simulink model "uwb_1"  (R2025a)
settings: Solver=VariableStepAuto  StartTime=0.0  StopTime=5e-08  RelTol=1e-3
undefined symbols (not defined in the file or in its folder): dspblkCoreblockFVToolHelper, gcbh
libraries: commdigbbndpm3 x2, dspfiltersrcs x2, dspsigops x2, simulink_extras x1, dspfdesign x1, simulink x1, commrfcorlib x1
settings Model: Creator=IWMAI  LastModifiedBy=IWMAI

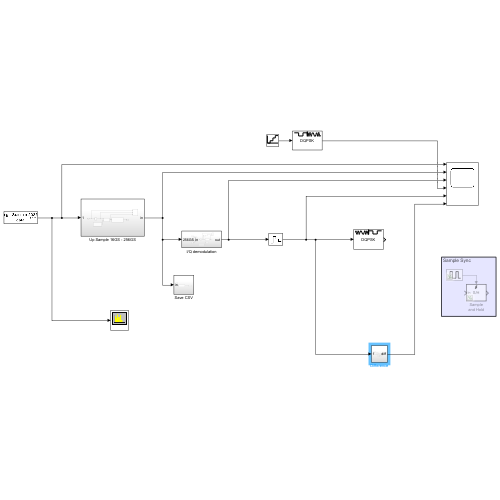
[thumbnail: Simulink's stored preview of the top-level diagram]
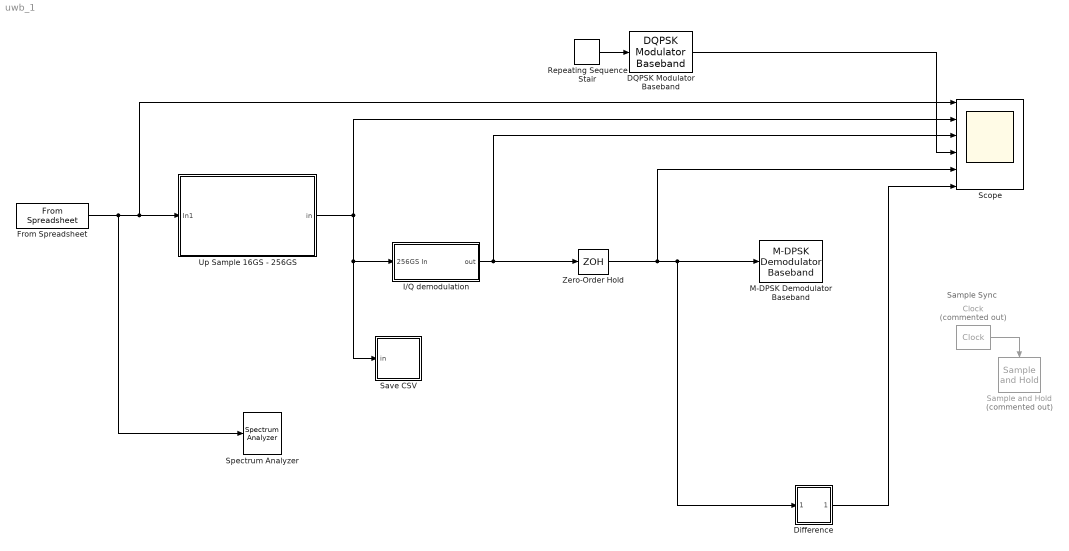
== system uwb_1 ==
  note: Sample Sync
  Clock : simulink_extras/Flip Flops/Clock  Commented=on  period=512.95 / 256e9
  DQPSK Modulator Baseband : commdigbbndpm3/DQPSK Modulator Baseband  InType=Integer  Enc=Gray  Ph=pi/4  outDtype=double
  Difference : Subsystem
  From Spreadsheet : FromSpreadsheet  FileName=C:\Users\IWMAI\University of Toronto\Yu Huang - Summer-2025-sharted\Yongkang\v3_250617\csv\data.csv  SheetName=data  OutDataTypeStr=double  SampleTime=6.25e-11
  I/Q demodulation : Subsystem
  M-DPSK Demodulator Baseband : commdigbbndpm3/M-DPSK Demodulator Baseband  M=4  OutType=Integer  Dec=Gray  Ph=pi/8  outDtype1=Inherit via internal rule  outDtype2=Inherit via internal rule
  Repeating Sequence Stair : simulink/Sources/Repeating Sequence Stair  OutValues=[0 1 2 3].'  tsamp=512.95 / 256e9  OutMin=[]  OutMax=[]  OutDataTypeStr=double  OutputDataTypeScalingMode=double  OutDataType=fixdt(0,8)  ConRadixGroup=Best Precision: Vector-wise  OutScaling=2^-12
  Sample and Hold : dspsigops/Sample and Hold  Commented=on  trig=Rising edge  initCond=0  latchinput=off
  Save CSV : Subsystem
  Scope : Scope  NumInputPorts=6
      settings: ActiveDisplayYMinimum=-0.1766463393208148  ActiveDisplayYMaximum=0.16150855826432609
  Spectrum Analyzer : SpectrumAnalyzer  WindowPosition=[624.000000,326.000000,800.000000,500.000000,]  ScopeFrameLocation=window  WindowInvariantSamplesPerUpdate=on  YLimits=[-72.7658 4.4718]
      settings: OpenAtSimulationStart=off
  Up Sample 16GS - 256GS : Subsystem
  Zero-Order Hold : ZeroOrderHold  SampleTime=512.95 / 256e9
  wires:
  From Spreadsheet/1 -> Spectrum Analyzer/1, Up Sample 16GS - 256GS/1(In1), Scope/1
  Up Sample 16GS - 256GS/1(in) -> Save CSV/1(in), I/Q demodulation/1(256GS In), Scope/2
  I/Q demodulation/1(out) -> Zero-Order Hold/1, Scope/3
  Zero-Order Hold/1 -> Scope/5, Difference/1(In1), M-DPSK Demodulator Baseband/1
  Clock/1 -> Sample and Hold/Trigger
  Repeating Sequence Stair/1 -> DQPSK Modulator Baseband/1
  DQPSK Modulator Baseband/1 -> Scope/4
  Difference/1(diff) -> Scope/6

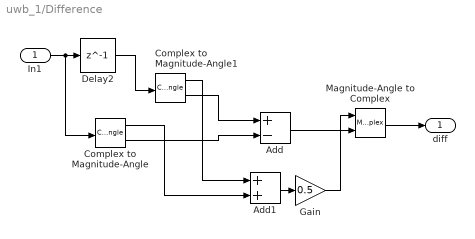
== system uwb_1/Difference ==
  In1 : Inport
  Add : Sum  Inputs=+-
  Add1 : Sum
  Complex to Magnitude-Angle : ComplexToMagnitudeAngle
  Complex to Magnitude-Angle1 : ComplexToMagnitudeAngle
  Delay2 : Delay  DelayLength=1
  Gain : Gain  Gain=0.5
  Magnitude-Angle to Complex : MagnitudeAngleToComplex
  diff : Outport
  wires:
  Gain/1 -> Magnitude-Angle to Complex/1
  Complex to Magnitude-Angle1/2 -> Add/1
  Add1/1 -> Gain/1
  Add/1 -> Magnitude-Angle to Complex/2
  Complex to Magnitude-Angle/2 -> Add/2
  Magnitude-Angle to Complex/1 -> diff/1
  Complex to Magnitude-Angle/1 -> Add1/2
  Complex to Magnitude-Angle1/1 -> Add1/1
  Delay2/1 -> Complex to Magnitude-Angle1/1
  In1/1 -> Delay2/1, Complex to Magnitude-Angle/1

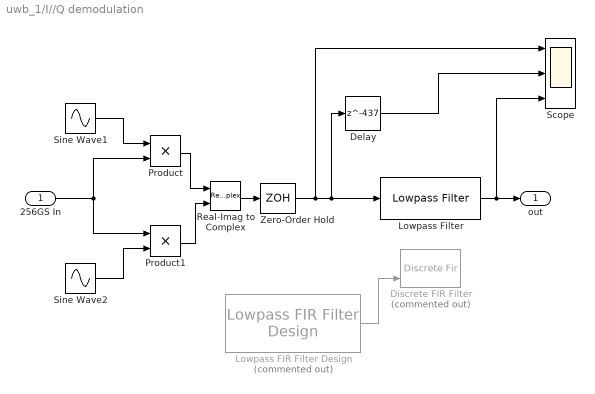
== system uwb_1/I//Q demodulation ==
  256GS In : Inport
  Delay : Delay  DelayLength=437
  Discrete FIR Filter : DiscreteFir  Commented=on  LoadFcn=dspblkCoreblockFVToolHelper(gcbh,'load');  CoefSource=Input port
      settings: CopyFcn=dspblkCoreblockFVToolHelper(gcbh,'copy');  DeleteFcn=dspblkCoreblockFVToolHelper(gcbh,'close');  ModelCloseFcn=dspblkCoreblockFVToolHelper(gcbh,'close');  PreSaveFcn=dspblkCoreblockFVToolHelper(gcbh,'presave');  PostSaveFcn=dspblkCoreblockFVToolHelper(gcbh,'postsave');  CloseFcn=dspblkCoreblockFVToolHelper(gcbh,'close');  InputPortMap=u0,u1
  Lowpass FIR Filter Design : dspfiltersrcs/Lowpass FIR Filter Design  Commented=on  SmoothParameters=off  SmoothingFactor=0.6  FilterOrderPort=off  FilterOrder=100  MaxOrder=100  CutoffFrequencyPort=off  CutoffFrequency=1/256e9  Window=Hann  SidelobeAttenuationPort=off  SidelobeAttenuation=60  KaiserWindowParameterPort=off  KaiserWindowParameter=.5  OutputDataType=double  SampleTime=1/256e9  SimulateUsing=Interpreted execution
      settings: LibrarySourceBlock=dspfdesign/Lowpass FIR Filter Design
  Lowpass Filter : dspfdesign/Lowpass Filter  FilterType=FIR  DesignForMinimumOrder=on  FilterOrder=50  PassbandFrequency=1/128  StopbandFrequency=1/64  PassbandRipple=0.1  StopbandAttenuation=80  SampleRateMode=Use normalized frequency (0 to 1)  SampleRate=44100  SimulateUsing=Interpreted execution  roundingMode=Floor  coeffsDataTypeStr=fixdt(1,16)
  Product : Product
  Product1 : Product
  Real-Imag to Complex : RealImagToComplex
  Scope : Scope  NumInputPorts=3
      settings: ActiveDisplayYMinimum=-6.0977483388597946  ActiveDisplayYMaximum=7.578935112423169  DataLoggingVariableName=ScopeData2
  Sine Wave1 : Sin  Frequency=2 * pi * 3.75e9  Phase=pi/2  SampleTime=0
  Sine Wave2 : Sin  Frequency=2 * pi * 3.75e9  SampleTime=0
  Zero-Order Hold : ZeroOrderHold  SampleTime=1/256e9
  out : Outport
  wires:
  256GS In/1 -> Product/2, Product1/1
  Sine Wave2/1 -> Product1/2
  Sine Wave1/1 -> Product/1
  Product/1 -> Real-Imag to Complex/1
  Product1/1 -> Real-Imag to Complex/2
  Lowpass FIR Filter Design/1 -> Discrete FIR Filter/2
  Lowpass Filter/1 -> Scope/3, out/1
  Real-Imag to Complex/1 -> Zero-Order Hold/1
  Zero-Order Hold/1 -> Scope/1, Delay/1, Lowpass Filter/1
  Delay/1 -> Scope/2

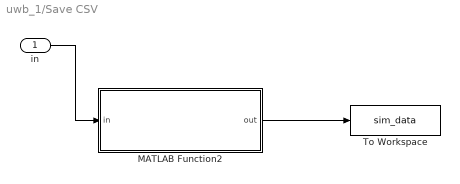
== system uwb_1/Save CSV ==
  in : Inport
  MATLAB Function2 : MATLAB Function  TreatAsAtomicUnit=on
  To Workspace : ToWorkspace  VariableName=sim_data  SaveFormat=Timeseries  SampleTime=-1
  wires:
  MATLAB Function2/1(out) -> To Workspace/1
  in/1 -> MATLAB Function2/1(in)

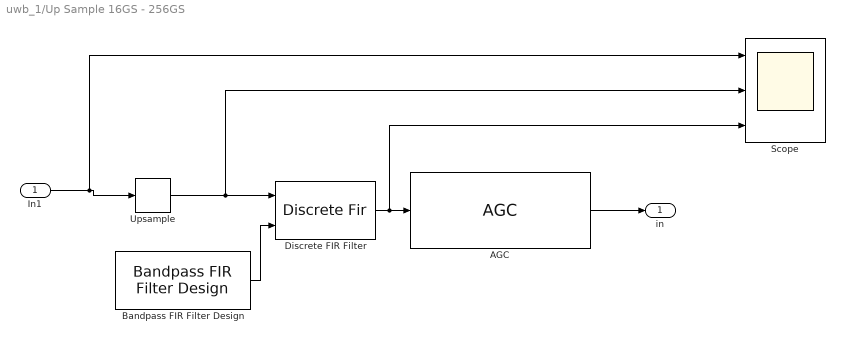
== system uwb_1/Up Sample 16GS - 256GS ==
  In1 : Inport
  AGC : commrfcorlib/AGC  LegacyMode=off  DetectorMethod=Rectifier  LoopMethod=Linear  UpdatePeriod=100  StepSize=0.1  AdaptationStepSize=0.01  DesiredOutputPower=1  AveragingLength=512  MaximumGain=30  MaxPowerGain=60  GainOutputPort=off  InputPowerOutputPort=off  SimulateUsing=Interpreted execution
  Bandpass FIR Filter Design : dspfiltersrcs/Bandpass FIR Filter Design  SmoothParameters=off  SmoothingFactor=0.6  FilterOrderPort=off  FilterOrder=100  MaxOrder=100  CenterFrequencyPort=off  CenterFrequency=1/64  BandwidthPort=off  Bandwidth=0.01  Window=Hann  SidelobeAttenuationPort=off  SidelobeAttenuation=60  KaiserWindowParameterPort=off  KaiserWindowParameter=.5  OutputDataType=double  SampleTime=256e9  SimulateUsing=Interpreted execution
      settings: LibrarySourceBlock=dspfdesign/Bandpass FIR Filter Design
  Discrete FIR Filter : DiscreteFir  LoadFcn=dspblkCoreblockFVToolHelper(gcbh,'load');  CoefSource=Input port
      settings: CopyFcn=dspblkCoreblockFVToolHelper(gcbh,'copy');  DeleteFcn=dspblkCoreblockFVToolHelper(gcbh,'close');  ModelCloseFcn=dspblkCoreblockFVToolHelper(gcbh,'close');  PreSaveFcn=dspblkCoreblockFVToolHelper(gcbh,'presave');  PostSaveFcn=dspblkCoreblockFVToolHelper(gcbh,'postsave');  CloseFcn=dspblkCoreblockFVToolHelper(gcbh,'close');  InputPortMap=u0,u1
  Scope : Scope  NumInputPorts=3
      settings: ActiveDisplayYMinimum=-0.1766463393208148  ActiveDisplayYMaximum=0.16150855826432609
  Upsample : dspsigops/Upsample  FactorSource=Dialog parameter  N=16  Nmax=16  phase=0  RateOptions=Allow multirate processing  ic=0  mode=Unused parameter value
      settings: LibrarySourceBlock=dsphdlsupportsigops/Upsample
  in : Outport
  wires:
  Upsample/1 -> Scope/2, Discrete FIR Filter/1
  Discrete FIR Filter/1 -> Scope/3, AGC/1
  AGC/1 -> in/1
  Bandpass FIR Filter Design/1 -> Discrete FIR Filter/2
  In1/1 -> Scope/1, Upsample/1

== matlab function uwb_1/Save CSV/MATLAB Function2 ==
  data: in input; out output
function out = save_csv(in)
%#codegen
% This function processes one sample at a time.
% To store data across simulation steps, you need to use persistent variables.

persistent data_buffer;
persistent index_counter;

if isempty(data_buffer)
    % Initialize buffer and counter when simulation starts or resets
    data_buffer = zeros(0, 2); % Column 1 for index, Column 2 for data
    index_counter = 0;
end

% Increment index and store current sample
index_counter = index_counter + 1;
data_buffer = [data_buffer; index_counter, in];

% Output the current sample (or anything else you need downstream)
out = in;

% You can add logic here to write to CSV periodically,
% but it's generally better to do it after simulation.
% For this method, we'll let 'To Workspace' handle saving.

% At the end of simulation, the persistent variables will be cleared unless
% you explicitly save them or access them from the base workspace.
% For 'To Workspace' method, it's about the *output* of this block.
end
